simulink model "untitled1"  (R2018b)
settings: Solver=VariableStepAuto  StartTime=0.0  StopTime=5  RelTol=1e-3
settings Model: Creator=nhat  LastModifiedBy=nhat

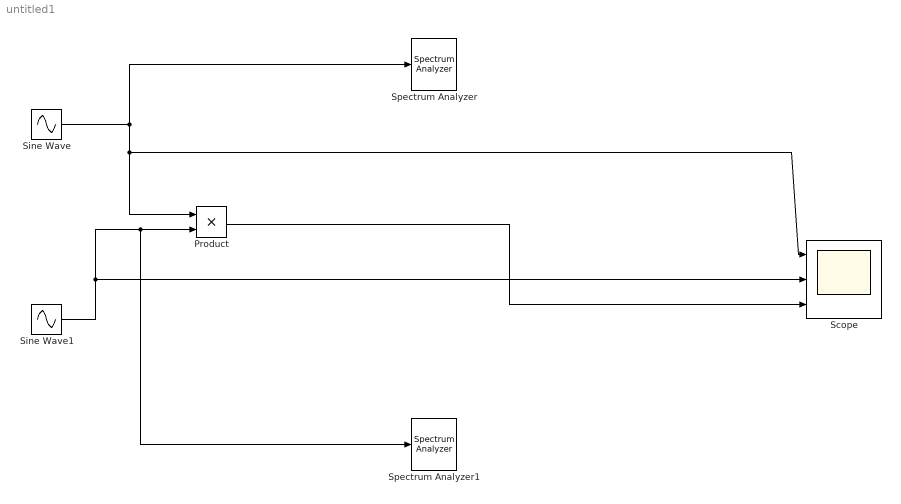
== system untitled1 ==
  Product : Product
  Scope : Scope  NumInputPorts=3
  Sine Wave : Sin  Frequency=1000*2*pi  SampleTime=1/400000
  Sine Wave1 : Sin  Frequency=10000*2*pi  SampleTime=1/400000
  Spectrum Analyzer : SpectrumAnalyzer
  Spectrum Analyzer1 : SpectrumAnalyzer
  wires:
  Sine Wave/1 -> Product/1, Scope/1, Spectrum Analyzer/1
  Sine Wave1/1 -> Spectrum Analyzer1/1, Product/2, Scope/2
  Product/1 -> Scope/3
